simulink model "simu"  (Simulink 8.5)
settings: Solver=ode45  StartTime=0.0  StopTime=10  RelTol=1e-3
values from neighbouring files (symbols this model uses):
  CoMxinit = ( c1+c2+c3+c4+c5 )/M    [init.m]
  K = 10    [init.m]
  Kp = 2    [init.m]
  tau = 0.1    [init.m]
  theta1 = pi/2    (= 1.57079632679)    [init.m]
  theta2 = -pi/2    (= -1.57079632679)    [init.m]
  theta3 = pi/2    (= 1.57079632679)    [init.m]
  theta4 = 3*pi/4    (= 2.35619449019)    [init.m]
  theta5 = -pi/2    (= -1.57079632679)    [init.m]
settings Model: Creator=msanchez04  LastModifiedBy=Michael
settings DebuggingCC: SolverPrmCheckMsg=warning  FcnCallInpInsideContextMsg=EnableAllAsWarning

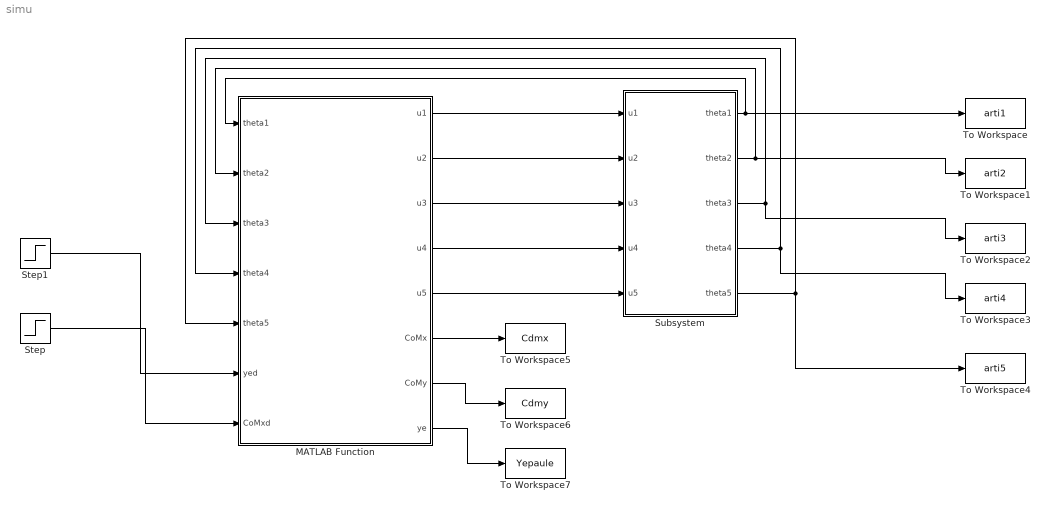
== system simu ==
  MATLAB Function : MATLAB Function  TreatAsAtomicUnit=on
  Step : Step  Before=CoMxinit  After=0  SampleTime=0
  Step1 : Step  Before=1.1  After=1.7  SampleTime=0
  Subsystem : Subsystem
  To Workspace : ToWorkspace  VariableName=arti1  SaveFormat=Timeseries  SampleTime=-1
  To Workspace1 : ToWorkspace  VariableName=arti2  SaveFormat=Timeseries  SampleTime=-1
  To Workspace2 : ToWorkspace  VariableName=arti3  SaveFormat=Timeseries  SampleTime=-1
  To Workspace3 : ToWorkspace  VariableName=arti4  SaveFormat=Timeseries  SampleTime=-1
  To Workspace4 : ToWorkspace  VariableName=arti5  SaveFormat=Timeseries  SampleTime=-1
  To Workspace5 : ToWorkspace  VariableName=Cdmx  SaveFormat=Timeseries  SampleTime=-1
  To Workspace6 : ToWorkspace  VariableName=Cdmy  SaveFormat=Timeseries  SampleTime=-1
  To Workspace7 : ToWorkspace  VariableName=Yepaule  SaveFormat=Timeseries  SampleTime=-1
  wires:
  MATLAB Function/1(u1) -> Subsystem/1(u1)
  MATLAB Function/2(u2) -> Subsystem/2(u2)
  MATLAB Function/3(u3) -> Subsystem/3(u3)
  MATLAB Function/4(u4) -> Subsystem/4(u4)
  MATLAB Function/5(u5) -> Subsystem/5(u5)
  Subsystem/1(theta1) -> To Workspace/1, MATLAB Function/1(theta1)
  Subsystem/2(theta2) -> To Workspace1/1, MATLAB Function/2(theta2)
  Subsystem/3(theta3) -> To Workspace2/1, MATLAB Function/3(theta3)
  Subsystem/4(theta4) -> To Workspace3/1, MATLAB Function/4(theta4)
  Subsystem/5(theta5) -> To Workspace4/1, MATLAB Function/5(theta5)
  Step1/1 -> MATLAB Function/6(yed)
  Step/1 -> MATLAB Function/7(CoMxd)
  MATLAB Function/6(CoMx) -> To Workspace5/1
  MATLAB Function/7(CoMy) -> To Workspace6/1
  MATLAB Function/8(ye) -> To Workspace7/1

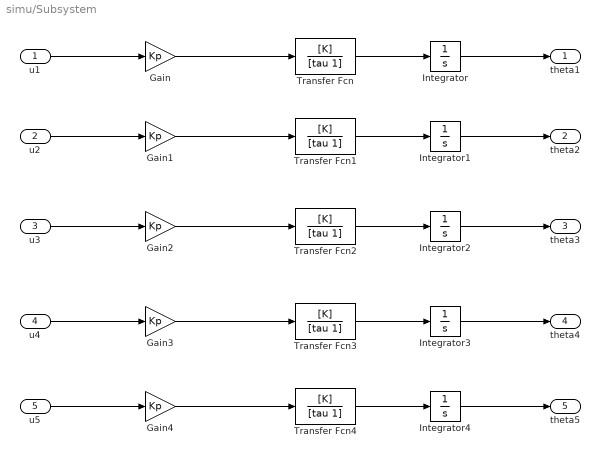
== system simu/Subsystem ==
  u1 : Inport
  u2 : Inport  Port=2
  u3 : Inport  Port=3
  u4 : Inport  Port=4
  u5 : Inport  Port=5
  Gain{,1..4} (5 alike) : Gain  Gain=Kp
  Integrator : Integrator  InitialCondition=theta1
  Integrator1 : Integrator  InitialCondition=theta2
  Integrator2 : Integrator  InitialCondition=theta3
  Integrator3 : Integrator  InitialCondition=theta4
  Integrator4 : Integrator  InitialCondition=theta5
  Transfer Fcn{,1..4} (5 alike) : TransferFcn  Numerator=[K]  Denominator=[tau 1]
  theta1 : Outport
  theta2 : Outport  Port=2
  theta3 : Outport  Port=3
  theta4 : Outport  Port=4
  theta5 : Outport  Port=5
  wires:
  Transfer Fcn/1 -> Integrator/1
  Transfer Fcn1/1 -> Integrator1/1
  Transfer Fcn2/1 -> Integrator2/1
  Transfer Fcn3/1 -> Integrator3/1
  Transfer Fcn4/1 -> Integrator4/1
  Integrator/1 -> theta1/1
  u1/1 -> Gain/1
  Integrator1/1 -> theta2/1
  u2/1 -> Gain1/1
  Integrator2/1 -> theta3/1
  u3/1 -> Gain2/1
  Integrator3/1 -> theta4/1
  u4/1 -> Gain3/1
  Integrator4/1 -> theta5/1
  u5/1 -> Gain4/1
  Gain/1 -> Transfer Fcn/1
  Gain1/1 -> Transfer Fcn1/1
  Gain2/1 -> Transfer Fcn2/1
  Gain3/1 -> Transfer Fcn3/1
  Gain4/1 -> Transfer Fcn4/1

== matlab function MATLAB Function ==
  data: theta1 input double; u1 output double; u2 output double; u3 output double; u4 output double; u5 output double; theta2 input double; theta3 input double; theta4 input double; theta5 input double; yed input double; CoMxd input double; CoMx output double; CoMy output double; ye output double
function [u1, u2, u3, u4, u5, CoMx, CoMy, ye] = fcn(theta1, theta2, theta3, theta4, theta5, yed, CoMxd)

% Variables
m1 = 15;
m2 = 25;
m3 = 35;
m4 = 10;
m5 = 5;

l1 = 0.4;
l2 = 0.6;
l3 = 0.7;
l4 = 0.6;
l5 = 0.35;
lbase = 0.3;

% Centre de masse suivant X (CoMx)
M = m1+m2+m3+m4+m5;

cx1 = 0.5*l1*cos(theta1)*m1;
cx2 = ( l1*cos(theta1)+0.5*l2*cos(theta1+theta2) )*m2;
cx3 = ( l1*cos(theta1)+l2*cos(theta1+theta2)+0.5*l3*cos(theta1+theta2+theta3) )*m3;
cx4 = ( l1*cos(theta1)+l2*cos(theta1+theta2)+l3*cos(theta1+theta2+theta3)+0.5*l4*cos(theta1+theta2+theta3+theta4) )*m4;
cx5 = ( l1*cos(theta1)+l2*cos(theta1+theta2)+l3*cos(theta1+theta2+theta3)+l4*cos(theta1+theta2+theta3+theta4)+0.5*l5*cos(theta1+theta2+theta3+theta4+theta5) )*m5;

cy1 = 0.5*l1*sin(theta1)*m1;
cy2 = ( l1*sin(theta1)+0.5*l2*sin(theta1+theta2) )*m2;
cy3 = ( l1*sin(theta1)+l2*sin(theta1+theta2)+0.5*l3*sin(theta1+theta2+theta3) )*m3;
cy4 = ( l1*sin(theta1)+l2*sin(theta1+theta2)+l3*sin(theta1+theta2+theta3)+0.5*l4*sin(theta1+theta2+theta3+theta4) )*m4;
cy5 = ( l1*sin(theta1)+l2*sin(theta1+theta2)+l3*sin(theta1+theta2+theta3)+l4*sin(theta1+theta2+theta3+theta4)+0.5*l5*sin(theta1+theta2+theta3+theta4+theta5) )*m5;

CoMx = ( cx1+cx2+cx3+cx4+cx5 )/M;
CoMy = ( cy1+cy2+cy3+cy4+cy5 )/M;

% Position de l'epaule suivant Y (ye)
ye = l1*sin(theta1)+l2*sin(theta1+theta2)+l3*sin(theta1+theta2+theta3);

% Jacobiennes Jcom (CoMx) et Je (ye)
j1 = -l1*sin(theta1)*( 0.5*m1+m2+m3+m4+m5) - l2*sin(theta1+theta2)*( 0.5*m2+m3+m4+m5) - l3*sin(theta1+theta2+theta3)*( 0.5*m3+m4+m5) - l4*sin(theta1+theta2+theta3+theta4)*( 0.5*m4+m5) - l5*sin(theta1+theta2+theta3+theta4+theta5)*0.5*m5;
j2 = -l2*sin(theta1+theta2)*( 0.5*m2+m3+m4+m5) - l3*sin(theta1+theta2+theta3)*( 0.5*m3+m4+m5) - l4*sin(theta1+theta2+theta3+theta4)*( 0.5*m4+m5) - l5*sin(theta1+theta2+theta3+theta4+theta5)*0.5*m5;
j3 = -l3*sin(theta1+theta2+theta3)*( 0.5*m3+m4+m5) - l4*sin(theta1+theta2+theta3+theta4)*( 0.5*m4+m5) - l5*sin(theta1+theta2+theta3+theta4+theta5)*0.5*m5;
j4 = -l4*sin(theta1+theta2+theta3+theta4)*( 0.5*m4+m5) - l5*sin(theta1+theta2+theta3+theta4+theta5)*0.5*m5;
j5 = -l5*sin(theta1+theta2+theta3+theta4+theta5)*0.5*m5;

Jcom = [j1 j2 j3 j4 j5];

Je = [l1*cos(theta1)+l2*cos(theta1+theta2)+l3*cos(theta1+theta2+theta3), l2*cos(theta1+theta2)+l3*cos(theta1+theta2+theta3), l3*cos(theta1+theta2+theta3), 0, 0];

%% Erreurs
err_com = CoMxd - CoMx;
err_ye = yed - ye;

I = eye(5);
Jey = Je*(I - pinv(Jcom)*Jcom);

err_theta = pinv(Jcom)*err_com + (I - pinv(Jcom)*Jcom)*pinv(Jey)*(err_ye - Je*pinv(Jcom)*err_com);

u1 = err_theta(1);
u2 = err_theta(2);
u3 = err_theta(3);
u4 = err_theta(4);
u5 = err_theta(5);
